simulink subsystem "wheelSpeed"  (R2022b)
settings: Solver=VariableStepAuto  StartTime=0.0  StopTime=10.0  RelTol=1e-3
libraries: Raptor_lib x4, wheelSpeed_lib x4
settings Model: Creator=serga  LastModifiedBy=serga

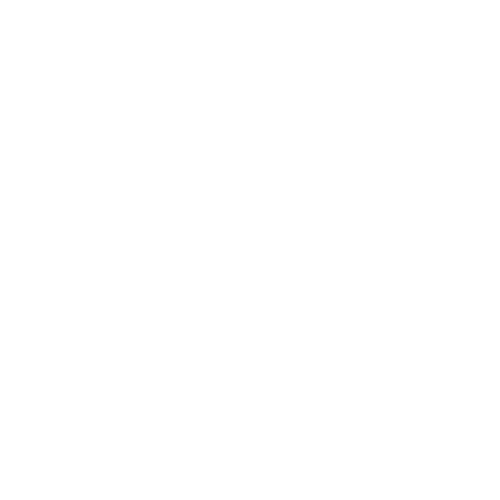
[thumbnail: Simulink's stored preview of the top-level diagram]
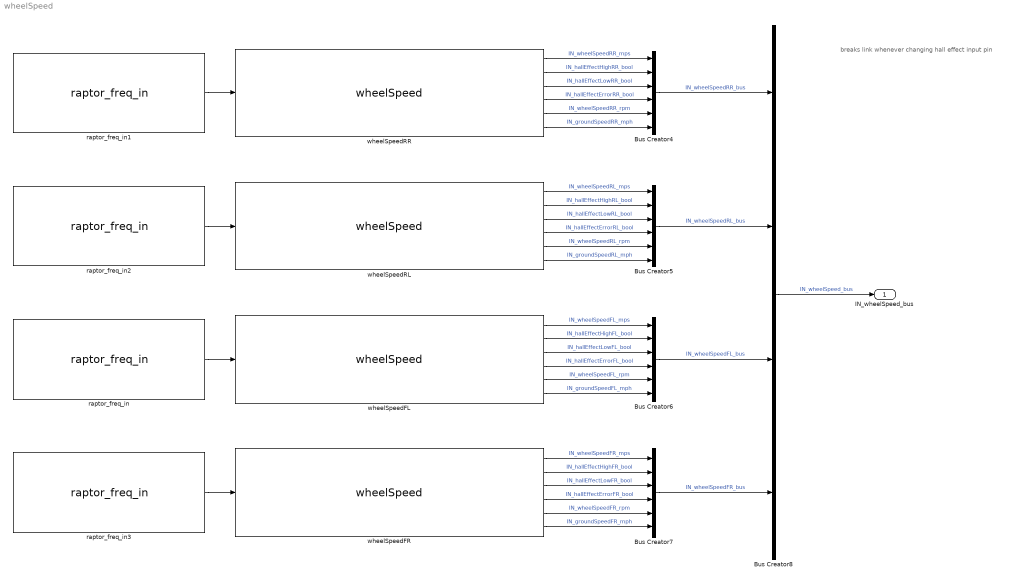
== system wheelSpeed ==
  note: breaks link whenever changing hall effect input pin
  Bus Creator{4..7} (4 alike) : BusCreator  Inputs=6
  Bus Creator8 : BusCreator  Inputs=4
  raptor_freq_in : Raptor_lib/Input & Output/raptor_freq_in  minFreq=1  resourceValues=INPUT41|INPUT42|INPUT43|INPUT44|INPUT45|(None)  resource=INPUT43  pullUDValues=[]  pullUD=[]  interfaceValues=[]  interface=[]  hasDuty=off  hasEdgeCount=off
      settings: SourceProductName=Raptor
  raptor_freq_in1 : Raptor_lib/Input & Output/raptor_freq_in  minFreq=1  resourceValues=INPUT41|INPUT42|INPUT43|INPUT44|INPUT45|(None)  resource=INPUT41  pullUDValues=[]  pullUD=[]  interfaceValues=[]  interface=[]  hasDuty=off  hasEdgeCount=off
      settings: SourceProductName=Raptor
  raptor_freq_in2 : Raptor_lib/Input & Output/raptor_freq_in  minFreq=1  resourceValues=INPUT41|INPUT42|INPUT43|INPUT44|INPUT45|(None)  resource=INPUT42  pullUDValues=[]  pullUD=[]  interfaceValues=[]  interface=[]  hasDuty=off  hasEdgeCount=off
      settings: SourceProductName=Raptor
  raptor_freq_in3 : Raptor_lib/Input & Output/raptor_freq_in  minFreq=1  resourceValues=INPUT41|INPUT42|INPUT43|INPUT44|INPUT45|(None)  resource=INPUT44  pullUDValues=[]  pullUD=[]  interfaceValues=[]  interface=[]  hasDuty=off  hasEdgeCount=off
      settings: SourceProductName=Raptor
  wheelSpeedFL : wheelSpeed_lib/wheelSpeed  pos='FL'
  wheelSpeedFR : wheelSpeed_lib/wheelSpeed  pos='FR'
  wheelSpeedRL : wheelSpeed_lib/wheelSpeed  pos='RL'
  wheelSpeedRR : wheelSpeed_lib/wheelSpeed  pos='RR'
  IN_wheelSpeed_bus : Outport
  wires:
  wheelSpeedRL/3 -> Bus Creator5/3  "IN_hallEffectLowRL_bool"
  wheelSpeedFL/5 -> Bus Creator6/5  "IN_wheelSpeedFL_rpm"
  wheelSpeedRL/2 -> Bus Creator5/2  "IN_hallEffectHighRL_bool"
  wheelSpeedFR/3 -> Bus Creator7/3  "IN_hallEffectLowFR_bool"
  wheelSpeedRR/1 -> Bus Creator4/1  "IN_wheelSpeedRR_mps"
  Bus Creator6/1 -> Bus Creator8/3  "IN_wheelSpeedFL_bus"
  wheelSpeedRL/1 -> Bus Creator5/1  "IN_wheelSpeedRL_mps"
  wheelSpeedRR/5 -> Bus Creator4/5  "IN_wheelSpeedRR_rpm"
  Bus Creator5/1 -> Bus Creator8/2  "IN_wheelSpeedRL_bus"
  wheelSpeedFR/2 -> Bus Creator7/2  "IN_hallEffectHighFR_bool"
  wheelSpeedFR/6 -> Bus Creator7/6  "IN_groundSpeedFR_mph"
  wheelSpeedFL/3 -> Bus Creator6/3  "IN_hallEffectLowFL_bool"
  wheelSpeedFL/1 -> Bus Creator6/1  "IN_wheelSpeedFL_mps"
  wheelSpeedRL/5 -> Bus Creator5/5  "IN_wheelSpeedRL_rpm"
  Bus Creator8/1 -> IN_wheelSpeed_bus/1  "IN_wheelSpeed_bus"
  wheelSpeedFL/2 -> Bus Creator6/2  "IN_hallEffectHighFL_bool"
  wheelSpeedRL/4 -> Bus Creator5/4  "IN_hallEffectErrorRL_bool"
  wheelSpeedFR/5 -> Bus Creator7/5  "IN_wheelSpeedFR_rpm"
  wheelSpeedRR/3 -> Bus Creator4/3  "IN_hallEffectLowRR_bool"
  Bus Creator7/1 -> Bus Creator8/4  "IN_wheelSpeedFR_bus"
  wheelSpeedRR/4 -> Bus Creator4/4  "IN_hallEffectErrorRR_bool"
  wheelSpeedFL/6 -> Bus Creator6/6  "IN_groundSpeedFL_mph"
  wheelSpeedRL/6 -> Bus Creator5/6  "IN_groundSpeedRL_mph"
  wheelSpeedFR/4 -> Bus Creator7/4  "IN_hallEffectErrorFR_bool"
  wheelSpeedFL/4 -> Bus Creator6/4  "IN_hallEffectErrorFL_bool"
  wheelSpeedRR/6 -> Bus Creator4/6  "IN_groundSpeedRR_mph"
  Bus Creator4/1 -> Bus Creator8/1  "IN_wheelSpeedRR_bus"
  wheelSpeedFR/1 -> Bus Creator7/1  "IN_wheelSpeedFR_mps"
  wheelSpeedRR/2 -> Bus Creator4/2  "IN_hallEffectHighRR_bool"
  raptor_freq_in1/1 -> wheelSpeedRR/1
  raptor_freq_in2/1 -> wheelSpeedRL/1
  raptor_freq_in/1 -> wheelSpeedFL/1
  raptor_freq_in3/1 -> wheelSpeedFR/1
